simulink model "doubleIt_sim"  (R2024a)
settings: Solver=VariableStepAuto  StartTime=0.0  StopTime=10.0  RelTol=1e-3
settings Model: Creator=miche  LastModifiedBy=miche
settings SFSimCC: SimCustomHeaderCode="#include \"doubleIt.h\""  SimUserSources=doubleIt.c

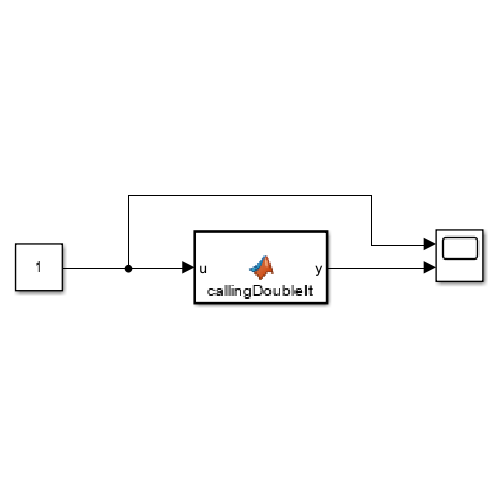
[thumbnail: Simulink's stored preview of the top-level diagram]
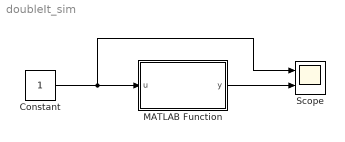
== system doubleIt_sim ==
  Constant : Constant
  MATLAB Function : MATLAB Function  TreatAsAtomicUnit=on
  Scope : Scope  NumInputPorts=2
  wires:
  Constant/1 -> Scope/1, MATLAB Function/1(u)
  MATLAB Function/1(y) -> Scope/2

== matlab function doubleIt_sim/MATLAB Function ==
  data: u input; y output
function y = callingDoubleIt(u)

y = 0.0;
y = coder.ceval("doubleIt",u);
